simulink model "Inverted_Pendulum_breach"  (R2020a)
settings: Solver=ode45  StartTime=0.0  StopTime=tspan(end)  RelTol=1e-3
model workspace: external: MATLAB File /home/nikhil/home/CSyn/src/pend_vars.m (data not in the file)
undefined symbols (not defined in the file or in its folder): b, g, I, l, m, M
settings Model: Creator=sansh  LastModifiedBy=nikhil
settings DataIOCC: ExternalInput=[t__, u__]  LoadExternalInput=on  SaveFormat=StructureWithTime
settings DebuggingCC: ArithmeticOperatorsInVariantConditions=warning
settings SFSimCC: SimUseLocalCustomCode=off  CustomCodeUndefinedFunction=UseInterfaceOnly
settings RTWCC: RTWUseLocalCustomCode=off
settings CodeAppCC: StateflowObjectComments=on
settings SimscapeCC: SimscapeNormalizeSystem=off

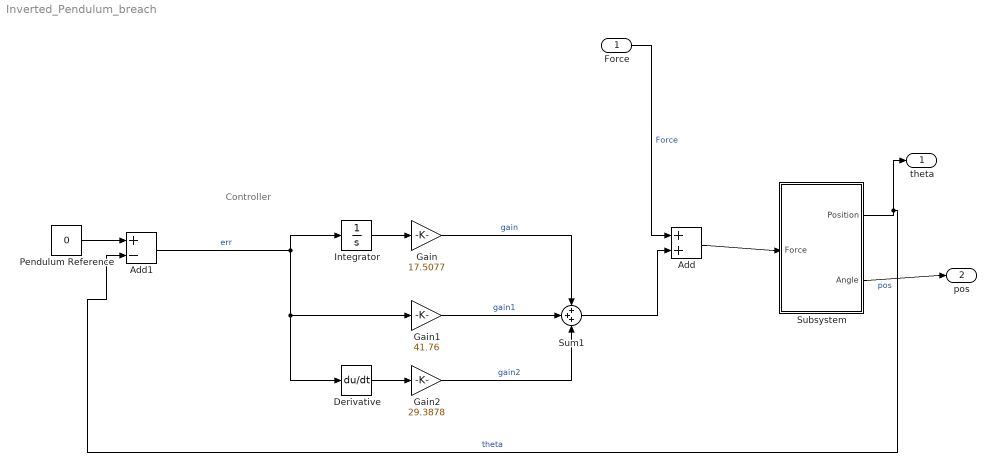
== system Inverted_Pendulum_breach ==
  note: Controller
  Force : Inport
  Add : Sum
  Add1 : Sum  Inputs=+-
  Derivative : Derivative
  Gain : Gain  Gain=17.5077
  Gain1 : Gain  Gain=41.76
  Gain2 : Gain  Gain=29.3878
  Integrator : Integrator
  Pendulum Reference : Constant  Value=0
  Subsystem : Subsystem
  Sum1 : Sum  Inputs=+++
  theta : Outport
  pos : Outport  Port=2
  wires:
  Add/1 -> Subsystem/1(Force)
  Subsystem/2(Angle) -> pos/1  "pos"
  Subsystem/1(Position) -> theta/1, Add1/2  "theta"
  Sum1/1 -> Add/2
  Pendulum Reference/1 -> Add1/1
  Force/1 -> Add/1  "Force"
  Gain/1 -> Sum1/1  "gain"
  Integrator/1 -> Gain/1
  Derivative/1 -> Gain2/1
  Gain1/1 -> Sum1/2  "gain1"
  Gain2/1 -> Sum1/3  "gain2"
  Add1/1 -> Integrator/1, Derivative/1, Gain1/1  "err"

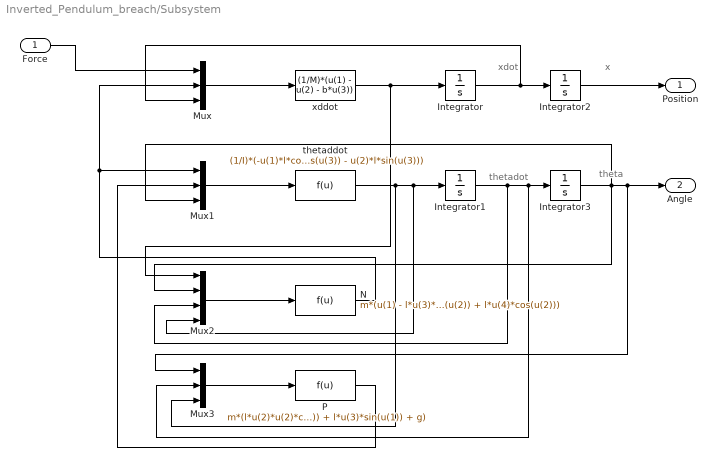
== system Inverted_Pendulum_breach/Subsystem ==
  note: theta
  note: x
  note: thetadot
  note: xdot
  Force : Inport
  Integrator : Integrator  ContinuousStateAttributes='xdot'
  Integrator1 : Integrator  ContinuousStateAttributes='thetadot'
  Integrator2 : Integrator  ContinuousStateAttributes='x'
  Integrator3 : Integrator  InitialCondition=pi  ContinuousStateAttributes='theta'
  Mux : Mux  Inputs=3
  Mux1 : Mux  Inputs=3
  Mux2 : Mux
  Mux3 : Mux  Inputs=3
  N : Fcn  Expr=m*(u(1) - l*u(3)*u(3)*sin(u(2)) + l*u(4)*cos(u(2)))
  P : Fcn  Expr=m*(l*u(2)*u(2)*cos(u(1)) + l*u(3)*sin(u(1)) + g)
  thetaddot : Fcn  Expr=(1/I)*(-u(1)*l*cos(u(3)) - u(2)*l*sin(u(3)))
  xddot : Fcn  Expr=(1/M)*(u(1) - u(2) - b*u(3))
  Position : Outport
  Angle : Outport  Port=2
  wires:
  Force/1 -> Mux/1
  Mux2/1 -> N/1
  Mux/1 -> xddot/1
  P/1 -> Mux1/2
  Mux3/1 -> P/1
  N/1 -> Mux1/1, Mux/2
  Mux1/1 -> thetaddot/1
  xddot/1 -> Mux2/1, Integrator/1
  Integrator2/1 -> Position/1
  thetaddot/1 -> Mux3/3, Mux2/4, Integrator1/1
  Integrator/1 -> Mux/3, Integrator2/1
  Integrator1/1 -> Mux2/3, Mux3/2, Integrator3/1
  Integrator3/1 -> Mux2/2, Mux1/3, Angle/1, Mux3/1
